simulink model "Gap_controller"  (Simulink 8.2)
settings: Solver=ode1  StartTime=0.0  StopTime=10.0  RelTol=1e-3
PostLoadFcn:
  | , if any(exist('dsrtsu_mdlpostloadfcn', 'file') == [2, 3, 6]), try dsrtsu_mdlpostloadfcn('Execute', bdroot); catch fprintf('Error in PostLoadFcn (dsrtsu_mdlpostloadfcn) for model "%s":\n %s\n', bdroot, lasterr); end, end,
settings Model: DSRTSU_INTERNAL_RTI_VER=450  DSRTSU_INTERNAL_RTI_TYPE=rti1401  DSRTSU_INTERNAL_RTIFPGA=40  Creator=Fang  LastModifiedBy=rushk1
settings DataIOCC: SignalLoggingSaveFormat=Dataset
settings OptimizationCC: InlineParams=on  ExpressionDepthLimit=128
settings DebuggingCC: FcnCallInpInsideContextMsg=EnableAllAsError  StateNameClashWarn=none
settings HardwareCC: ProdHWDeviceType=Generic->Unspecified (assume 32-bit Generic)  TargetIntDivRoundTo=Zero  TargetEndianess=BigEndian  TargetHWDeviceType=Generic->Custom
settings RTWCC: SystemTargetFile=rti1401.tlc  MakeCommand=make_rti  TemplateMakefile=rti1401.tmf  Description=dSPACE DS1401 Hardware Platform  ProcessScript=rti1401_make_rtw_hook
settings STFCustomTargetCC: CodeReplacementLibrary=ANSI_C  ParMdlRefBuildCompliant=on  GeneratePreprocessorConditionals=Disable all  MatFileLogging=on  SystemTargetFile=rti1401.tlc
settings GRTTargetCC: CompOptLevelCompliant=off  ConcurrentExecutionCompliant=off  ExtModeMexFile=noextcomm
settings CustomProperty: DataType=RTWOptions_EnumType_C__Program Files_dSPACE RCPHIL 2014-B_MATLAB_RTI_RTI1401_TLC_rti1401_1InitialSimState  Value=RUN
settings EnumStrPairs: String=RUN

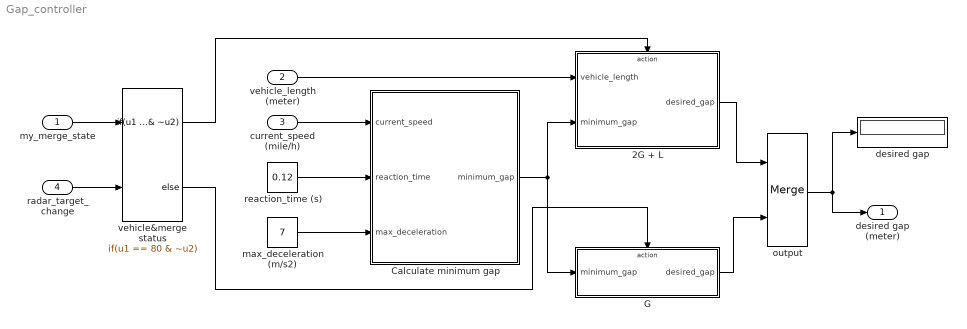
== system Gap_controller ==
  my_merge_state : Inport
  vehicle_length (meter) : Inport  Port=2
  current_speed (mile/h) : Inport  Port=3
  radar_target_change : Inport  Port=4  OutDataTypeStr=boolean
  2G + L : Subsystem  TreatAsAtomicUnit=on
  Calculate minimum gap : Subsystem
  G : Subsystem  TreatAsAtomicUnit=on
  desired gap : Display
  max_deceleration (m/s2) : Constant  Value=7
  output : Merge
  reaction_time (s) : Constant  Value=0.12
  vehicle&merge status : If  NumInputs=2  IfExpression=u1 == 80 & ~u2
  desired gap (meter) : Outport
  wires:
  reaction_time (s)/1 -> Calculate minimum gap/2(reaction_time)
  max_deceleration (m/s2)/1 -> Calculate minimum gap/3(max_deceleration)
  vehicle&merge status/1 -> 2G + L/Action
  vehicle&merge status/2 -> G/Action
  Calculate minimum gap/1(minimum_gap) -> 2G + L/2(minimum_gap), G/1(minimum_gap)
  2G + L/1(desired_gap) -> output/1
  G/1(desired_gap) -> output/2
  output/1 -> desired gap (meter)/1, desired gap/1
  vehicle_length (meter)/1 -> 2G + L/1(vehicle_length)
  current_speed (mile/h)/1 -> Calculate minimum gap/1(current_speed)
  my_merge_state/1 -> vehicle&merge status/1
  radar_target_change/1 -> vehicle&merge status/2

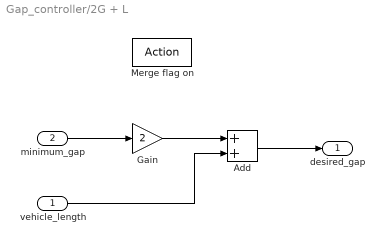
== system Gap_controller/2G + L ==
  vehicle_length : Inport
  minimum_gap : Inport  Port=2
  Merge flag on : ActionPort  ActionType=then
  Add : Sum
  Gain : Gain  Gain=2
  desired_gap : Outport
  wires:
  minimum_gap/1 -> Gain/1
  Gain/1 -> Add/1
  vehicle_length/1 -> Add/2
  Add/1 -> desired_gap/1

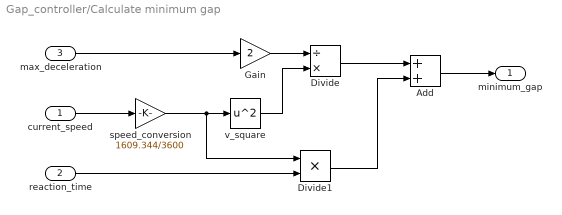
== system Gap_controller/Calculate minimum gap ==
  current_speed : Inport
  reaction_time : Inport  Port=2
  max_deceleration : Inport  Port=3
  Add : Sum
  Divide : Product  Inputs=/*
  Divide1 : Product  Inputs=**
  Gain : Gain  Gain=2
  speed_conversion : Gain  Gain=1609.344/3600
  v_square : Math  Operator=square  SaturateOnIntegerOverflow=on
  minimum_gap : Outport
  wires:
  Divide/1 -> Add/1
  Divide1/1 -> Add/2
  Add/1 -> minimum_gap/1
  Gain/1 -> Divide/1
  max_deceleration/1 -> Gain/1
  v_square/1 -> Divide/2
  reaction_time/1 -> Divide1/2
  current_speed/1 -> speed_conversion/1
  speed_conversion/1 -> Divide1/1, v_square/1

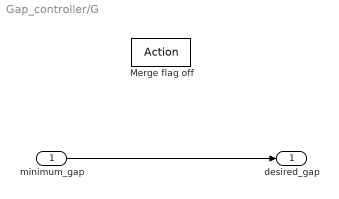
== system Gap_controller/G ==
  minimum_gap : Inport
  Merge flag off : ActionPort  ActionType=else
  desired_gap : Outport
  wires:
  minimum_gap/1 -> desired_gap/1
